simulink library "INT_CoETS_NTC"  (R2016b)
settings: Solver=VariableStepAuto  StartTime=0.0  StopTime=10.0  RelTol=1e-3
settings Model: Creator=Administrator  LastModifiedBy=Administrator

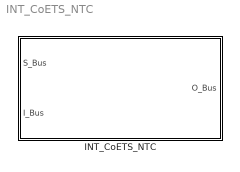
== system INT_CoETS_NTC ==
  INT_CoETS_NTC : Subsystem

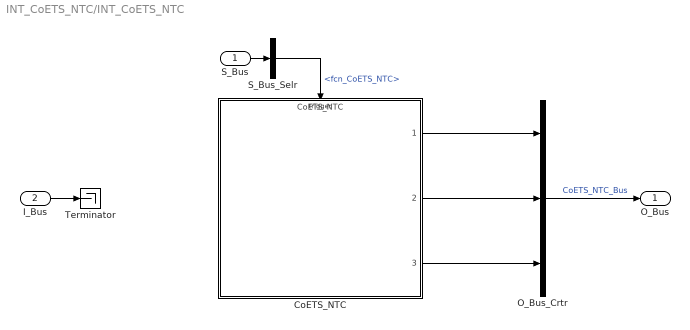
== system INT_CoETS_NTC/INT_CoETS_NTC ==
  S_Bus : Inport
  I_Bus : Inport  Port=2
  CoETS_NTC : ModelReference  ModelNameDialog=CoETS_NTC  SimulationMode=Normal  ModelReferenceVersion=1.7  TriggerPortName=function  TriggerPortTriggerType=function-call  TriggerPortStatesWhenEnabling=held
  O_Bus_Crtr : BusCreator  Inputs=3
  S_Bus_Selr : BusSelector  OutputSignals=fcn_CoETS_NTC
  Terminator : Terminator
  O_Bus : Outport
  wires:
  S_Bus_Selr/1 -> CoETS_NTC/Trigger  "<fcn_CoETS_NTC>"
  S_Bus/1 -> S_Bus_Selr/1
  I_Bus/1 -> Terminator/1
  O_Bus_Crtr/1 -> O_Bus/1  "CoETS_NTC_Bus"
  CoETS_NTC/1 -> O_Bus_Crtr/1
  CoETS_NTC/2 -> O_Bus_Crtr/2
  CoETS_NTC/3 -> O_Bus_Crtr/3
